simulink model "linear2D"  (Simulink 3.00)
settings: Solver=ode45  StartTime=0.0  StopTime=20  MaxStep=.01  RelTol=1e-3  AbsTol=1e-3
settings Model: SaveTime=off  SaveOutput=off  UnconnectedInputMsg=none  UnconnectedOutputMsg=none  UnconnectedLineMsg=none  InheritedTsInSrcMsg=none  LastModifiedBy=Administrator

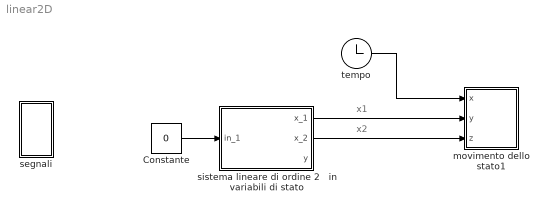
== system linear2D ==
  note: x1
  note: x2
  Constante : Constant  Value=0
  movimento dello stato1 : Subsystem  mask(grafico 3D){xlim=[0,20], ylim=[-pi 2*pi], zlim=[-3,3], view=[10 30]}
      mask prompts: xlim "t [min,max]:"; ylim "x1 [min,max]:"; zlim "x2 [min,max]:"; view "Orientamento:"
      mask help:
      | Movimento dello stato del sistema
      | Introdurre gli intervalli di rappresentazione del tempo e dello stato
      mask init:
      | st=-1;
      mask Help: This block can be used to explore limit cycles. Look at the m-file sfunxyz.m to see how it works.
      mask Display: plot(0,0,100,100,[12,91,91,12,12],[90,90,45,45,90],[51,57,65,75,80,79,75,67,60,54,51,48,42,34,28,27,31,42,51],[71,68,66,66,72,79,83,84,81,77,71,60,54,54,58,65,71,74,71])
  segnali : Subsystem
  sistema lineare di ordine 2   in variabili di stato : Subsystem  mask(2D state-space system ){A=[-1 0; 0 -1], B=[ 1; 1], C=[0 0], x0=[pi; 0]}
      mask prompts: A "2 by 2 dynamic matrix A:"; B "2 by 1 input matrix B:"; C "1 by 2 output matrix C:"; x0 "initial conditions x0:"
      mask Display: disp('dx/dt=Ax+Bu\n y=Cx             ')
  tempo : Clock
      settings: DisplayTime=off  Decimation=10
  wires:
  Constante/1 -> sistema lineare di ordine 2   in variabili di stato/1(in_1)
  tempo/1 -> movimento dello stato1/1(x)
  sistema lineare di ordine 2   in variabili di stato/1(x_1) -> movimento dello stato1/2(y)
  sistema lineare di ordine 2   in variabili di stato/2(x_2) -> movimento dello stato1/3(z)

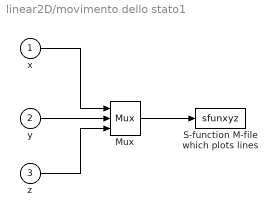
== system linear2D/movimento dello stato1 ==
  x : Inport  Port=1  PortWidth=-1  SampleTime=-1  DataType=auto
      settings: SignalType=auto
  y : Inport  Port=2  PortWidth=-1  SampleTime=-1  DataType=auto
      settings: SignalType=auto
  z : Inport  Port=3  PortWidth=-1  SampleTime=-1  DataType=auto
      settings: SignalType=auto
  Mux : Mux  Inputs=3
      settings: DisplayOption=none
  "S-function M-file which plots lines " : S-Function  FunctionName=sfunxyz  Parameters=xlim,ylim,zlim,view,st  PortCounts=[]  SFunctionModules=''
  wires:
  Mux/1 -> "S-function M-file which plots lines "/1
  x/1 -> Mux/1
  y/1 -> Mux/2
  z/1 -> Mux/3

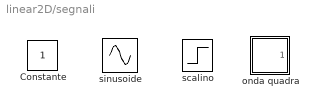
== system linear2D/segnali ==
  Constante : Constant  Value=1
  onda quadra : Subsystem  mask(Pulse Generator){@1=2, @2=1, @3=1, @4=0}
      mask prompts: @1 "Pulse period (secs):"; @2 "Pulse width:"; @3 "Pulse height:"; @4 "Pulse start time:"
      mask help: Pulse Generator.
      mask init:
      | Ts=@1; du=@2; ht=@3; stt=@4; ini=ones(length(ht),1); st1=rem(stt,Ts); st2=rem(stt+du,Ts);if(Ts<=1.2*du),ini=zeros(length(ht),1);end;
      mask Help: Pulse generator which ensures pulse\ntransitions are hit. Provides a vector of pulses when the height is entered as a vector.\nUnmask to see how it works.
      mask Display: plot(0,0,100,100,[90,75,75,60,60,35,35,20,20,10],[20,20,80,80,20,20,80,80,20,20])
  scalino : Step  Time=0  Before=0  After=1  SampleTime=-1
  sinusoide : Sin  Amplitude=1  Frequency=1  Phase=0  SampleTime=-1

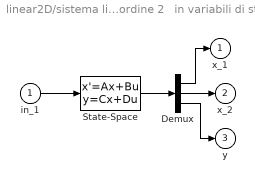
== system linear2D/sistema lineare di ordine 2   in variabili di stato ==
  in_1 : Inport  Port=1  PortWidth=-1  SampleTime=-1  DataType=auto
      settings: SignalType=auto
  Demux : Demux  Outputs=3
  State-Space : StateSpace  A=A  B=B  C=[1 0; 0 1; C]  D=[0 0 0]'  X0=x0
  x_1 : Outport  Port=1
  x_2 : Outport  Port=2
  y : Outport  Port=3
  wires:
  in_1/1 -> State-Space/1
  State-Space/1 -> Demux/1
  Demux/1 -> x_1/1
  Demux/2 -> x_2/1
  Demux/3 -> y/1

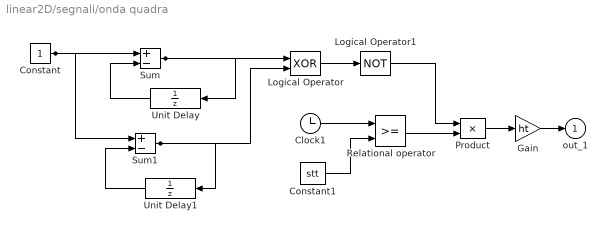
== system linear2D/segnali/onda quadra ==
  Clock1 : Clock
      settings: DisplayTime=off  Decimation=10
  Constant : Constant  Value=1
  Constant1 : Constant  Value=stt
  Gain : Gain  Gain=ht  SaturateOnIntegerOverflow=on
  Logical Operator : Logic  Operator=XOR  Inputs=2
  Logical Operator1 : Logic  Operator=NOT  Inputs=1
  Product : Product  Inputs=2  SaturateOnIntegerOverflow=on
  Relational operator : RelationalOperator  Operator=>=
  Sum : Sum  Inputs=+-  SaturateOnIntegerOverflow=on
  Sum1 : Sum  Inputs=+-  SaturateOnIntegerOverflow=on
  Unit Delay : UnitDelay  Orientation=left  X0=0  SampleTime=[Ts,st1]
  Unit Delay1 : UnitDelay  Orientation=left  X0=ini  SampleTime=[Ts,st2]
  out_1 : Outport  Port=1
  wires:
  Logical Operator1/1 -> Product/1
  Logical Operator/1 -> Logical Operator1/1
  Constant1/1 -> Relational operator/2
  Gain/1 -> out_1/1
  Product/1 -> Gain/1
  Relational operator/1 -> Product/2
  Clock1/1 -> Relational operator/1
  Unit Delay/1 -> Sum/2
  Unit Delay1/1 -> Sum1/2
  Constant/1 -> Sum/1, Sum1/1
  Sum/1 -> Unit Delay/1, Logical Operator/1
  Sum1/1 -> Unit Delay1/1, Logical Operator/2
